simulink model "mup_rmpcblock_demo_model_R2011b"  (Simulink 7.8)
settings: Solver=ode4  StartTime=0.0  StopTime=25  RelTol=1e-3
values from neighbouring files (symbols this model uses):
  A = model.A    [feas_init.m]    (also in mup_expand_rmpc_block_ws.m)
  B = model.B    [feas_init.m]    (also in mup_expand_rmpc_block_ws.m)
  C = model.C    [feas_init.m]    (also in mup_expand_rmpc_block_ws.m)
  nu = size(B{1},2)    [feas_init.m]    (also in mup_expand_rmpc_block_ws.m = problem.nu; mup_rmpcblock_demo.m; mup_sdp.m = problem.nu; rmpc_plot.m = size(data.u{1},1))
  nx = size(A{1},2)    [feas_init.m]    (also in mup_expand_rmpc_block_ws.m = problem.nx; mup_rmpcblock_demo.m; mup_sdp.m = problem.nx; rmpc_plot.m = size(data.x{1},1))
  ts = in(end)    [mup_rmpc_controller.m]    (also in mup_rmpc_counter.m = x(2); mup_rmpcblock_demo.m = 1; rmpc_plot.m = data.ts; rmpc_plot_r13b.m = data.ts)
  u_max = design.u_max    [feas_init.m]    (also in mup_expand_rmpc_block_ws.m; mup_rmpc_demo.m = [10]; mup_rmpcblock_demo.m = [10])
  Wu = design.Wu    [feas_init.m]    (also in mup_expand_rmpc_block_ws.m; mup_rmpc_demo.m = eye(1); mup_rmpcblock_demo.m = eye(1))
  Wx = design.Wx    [feas_init.m]    (also in mup_expand_rmpc_block_ws.m; mup_rmpc_demo.m = eye(2); mup_rmpcblock_demo.m = eye(2))
  x0 = design.x0    [mup_expand_rmpc_block_ws.m]    (also in mup_rmpc_demo.m = [3;0]; mup_rmpcblock_demo.m = [3;0])
  x_max = design.x_max    [feas_init.m]    (also in mup_expand_rmpc_block_ws.m; mup_rmpc_demo.m = [10;10]; mup_rmpcblock_demo.m = [10;10])
settings Model: Creator=oravec  LastModifiedBy=oravec
settings DataIOCC: SignalLoggingSaveFormat=Dataset
settings OptimizationCC: ExpressionDepthLimit=128
settings CodeAppCC: CustomSymbolStrType=$N$R$M_T
settings GRTTargetCC: TargetFunctionLibrary=C89/C90 (ANSI)

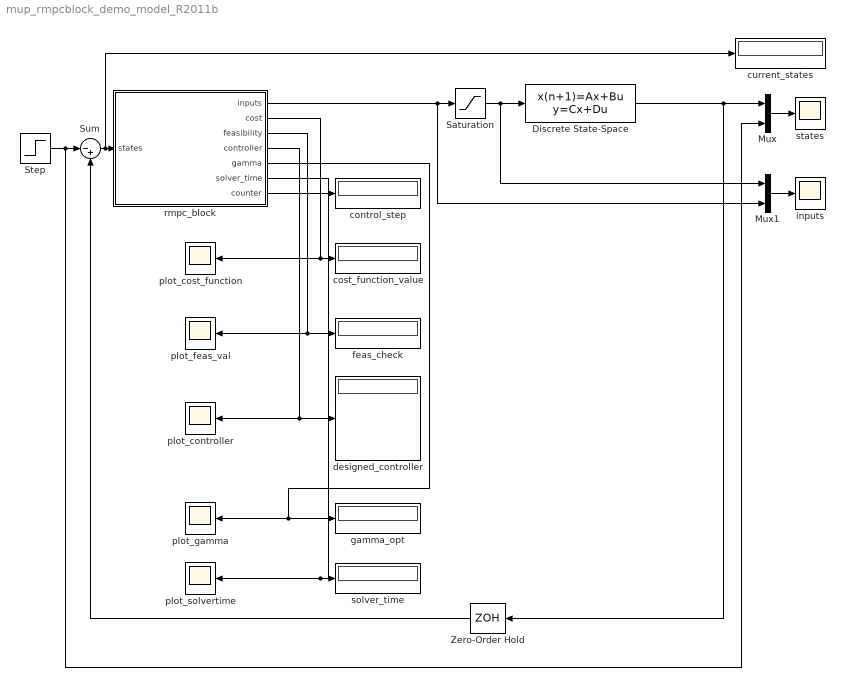
== system mup_rmpcblock_demo_model_R2011b ==
  Discrete State-Space : DiscreteStateSpace  A=A{vtx}  B=B{vtx}  C=C{vtx}  D=zeros(nx,nu)  X0=x0  SampleTime=ts
  Mux : Mux  Inputs=2
  Mux1 : Mux  Inputs=2
  Saturation : Saturate  UpperLimit=u_max  LowerLimit=-u_max
  Step : Step  Time=0  Before=zeros(nx,1)  After=zeros(nx,1)  SampleTime=0
  Sum : Sum  Inputs=|-+
  Zero-Order Hold : ZeroOrderHold  SampleTime=ts
  control_step : Display
  cost_function_value : Display
  current_states : Display
  designed_controller : Display
  feas_check : Display
  gamma_opt : Display
  inputs : Scope
      settings: YMin=-1.1  YMax=0.3  SaveName=data_u
  plot_controller : Scope
      settings: YMin=0  YMax=2  SaveName=f_des
  plot_cost_function : Scope
      settings: YMin=0  YMax=2  SaveName=cost
  plot_feas_val : Scope
      settings: YMin=0  YMax=2  SaveName=feas_val
  plot_gamma : Scope
      settings: YMin=0  YMax=2  SaveName=gamma_val
  plot_solvertime : Scope
      settings: YMin=0  YMax=2  SaveName=solvertime_val
  rmpc_block : Subsystem  Tag=rmpc_tag  mask(RMPC){rmpc_method=Kothare et al. (1996), opt_type=initial, chk_feas=on, feas_toler=-1e-6, x0=x0, A=A, B=B, C=C, Ts=ts, Wu=Wu, Wx=Wx, u_max=u_max, x_max=x_max, param=[], chk_soft_con=off, u_sl=[], y_sl=[], Wsu=[], Wsy=[], solver=MOSEK, vbs=Normal, vbsy=Silent}
      mask prompts: rmpc_method "Robust MPC Approach:"; opt_type "Optimization Problem Design:"; chk_feas "Feasibility Check (Disable to speed up control)"; feas_toler "Feasibility Tolerance: (Relevant, if Feasibility Check is enable)"; x0 "Initial Conditions of System States: x0"; A "System State Matrix: A"; B "System Input Matrix: B"; C "System Output Matrix: C"; Ts "Sampling Time: Ts"; Wu "Cost Function Weight of Inputs: Wu"; Wx "Cost Function Weight of States: Wx"; u_max "Symmetric Constraint on Control Input: u_max"; x_max "Symmetric Constraint on System Outputs: y_max"; param "Parameters:"; chk_soft_con "Consider Soft Constraints: chk_soft_con"; u_sl "Soft-constrained Control Inputs: u_sl"; y_sl "Soft-constrained System Outputs: y_sl"; Wsu "Weight of Soft-constrained Control Inputs: Wsu"; Wsy "Weight of Soft-constrained System Outputs: Wsy"; solver "SDP Solver:"; vbs "Verbose Mode:"; vbsy "YALMIP Verbose Mode:"
      mask help: Computes on-line robust MPC control inputs for a given state.
      mask init:
      | mup_rmpc_data
      | mup_rmpc_init(design,model,setup)
      mask Help: eval('mup_rmpc_help')
      mask StyleString: popup(Kothare et al. (1996)|Cuzzola et al. (2002)|Mao (2003)|Wan et al. (2003)|Cao et al. (2005)|Ding et al. (2007)|Li et al. (2008)|Huang et al. (2011)|Zhang et al. (2013)|NSO and ACIS|NSO and WACIS|NSO and SDLF|PDLF and ACIS|PDLF and WACIS|Kothare et al. (1996) - Soft-Con|Wan et al. (2003) - Soft-Con|Cao et al. (2005) - Soft-Con|NSO and ACIS - Soft-Con),popup(initial|reformulation),checkbox,edit,edit,edit,edit,edit,edit,edit,edit,edit,edit,edit,checkbox,edit,edit,edit,edit,popup(CSDP|DSDP|LMILAB|LOGDETPPA|MOSEK|PENBMI|PENLAB|PENSDP|SDPA|SDPLR|SDPT3|SDPNAL|SEDUMI),popup(Normal|Silent|Loud),popup(Silent|Loud)
      mask TabNameString: Robust MPC Configuration,Robust MPC Configuration,Robust MPC Configuration,Robust MPC Configuration,Robust MPC Configuration,Robust MPC Configuration,Robust MPC Configuration,Robust MPC Configuration,Robust MPC Configuration,Robust MPC Configuration,Robust MPC Configuration,Robust MPC Configuration,Robust MPC Configuration,Robust MPC Configuration,SOFT-CON,SOFT-CON,SOFT-CON,SOFT-CON,SOFT-CON,Setup,Setup,Setup
      mask Display:
      | disp('RMPC')
      | port_label('input',1,'states')
      | port_label('output',1,'inputs')
      | port_label('output',2,'cost')
      | port_label('output',3,'feasibility')
      | port_label('output',4,'controller')
      | port_label('output',5,'gamma')
      | port_label('output',6,'solver_time')
      | port_label('output',7,'counter')
  solver_time : Display
  states : Scope
      settings: YMin=-0.02  YMax=0.1  SaveName=data_x
  wires:
  rmpc_block/2(cost) -> plot_cost_function/1, cost_function_value/1
  Sum/1 -> rmpc_block/1(states), current_states/1
  Step/1 -> Mux/2, Sum/1
  Discrete State-Space/1 -> Mux/1, Zero-Order Hold/1
  Zero-Order Hold/1 -> Sum/2
  Mux/1 -> states/1
  Saturation/1 -> Discrete State-Space/1, Mux1/1
  rmpc_block/1(inputs) -> Saturation/1, Mux1/2
  Mux1/1 -> inputs/1
  rmpc_block/7(counter) -> control_step/1
  rmpc_block/3(feasibility) -> feas_check/1, plot_feas_val/1
  rmpc_block/4(controller) -> designed_controller/1, plot_controller/1
  rmpc_block/5(gamma) -> gamma_opt/1, plot_gamma/1
  rmpc_block/6(solver_time) -> plot_solvertime/1, solver_time/1

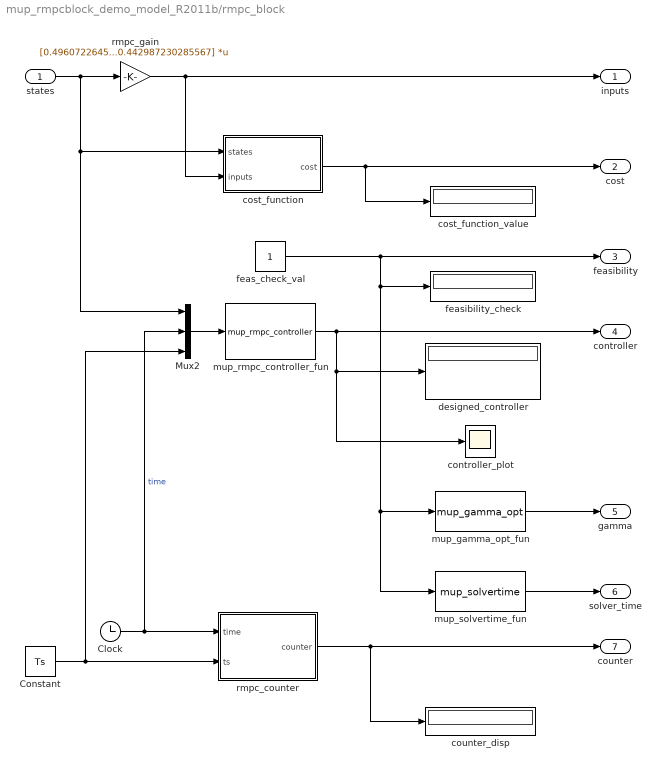
== system mup_rmpcblock_demo_model_R2011b/rmpc_block ==
  states : Inport
  Clock : Clock
  Constant : Constant  Value=Ts
  Mux2 : Mux  Inputs=3
  controller_plot : Scope
      settings: TimeRange=50  SaveName=rmpc_designed_controller  MaxDataPoints=50000
  cost_function : Subsystem
  cost_function_value : Display
  counter_disp : Display
  designed_controller : Display
  feas_check_val : Constant
  feasibility_check : Display
  mup_gamma_opt_fun : MATLABFcn  MATLABFcn=mup_gamma_opt
  mup_rmpc_controller_fun : MATLABFcn  MATLABFcn=mup_rmpc_controller
  mup_solvertime_fun : MATLABFcn  MATLABFcn=mup_solvertime
  rmpc_counter : Subsystem
  rmpc_gain : Gain  Tag=rmpc_gain_2013_3_25_11_17_59.8099  Gain=[0.496072264545493,0.442987230285567]  Multiplication=Matrix(K*u)
  inputs : Outport
  cost : Outport  Port=2
  feasibility : Outport  Port=3
  controller : Outport  Port=4
  gamma : Outport  Port=5
  solver_time : Outport  Port=6
  counter : Outport  Port=7
  wires:
  rmpc_gain/1 -> inputs/1, cost_function/2(inputs)
  states/1 -> rmpc_gain/1, Mux2/1, cost_function/1(states)
  cost_function/1(cost) -> cost_function_value/1, cost/1
  rmpc_counter/1(counter) -> counter_disp/1, counter/1
  Clock/1 -> rmpc_counter/1(time), Mux2/2  "time"
  Constant/1 -> rmpc_counter/2(ts), Mux2/3
  feas_check_val/1 -> feasibility/1, mup_solvertime_fun/1, mup_gamma_opt_fun/1, feasibility_check/1
  mup_rmpc_controller_fun/1 -> controller/1, designed_controller/1, controller_plot/1
  Mux2/1 -> mup_rmpc_controller_fun/1
  mup_gamma_opt_fun/1 -> gamma/1
  mup_solvertime_fun/1 -> solver_time/1

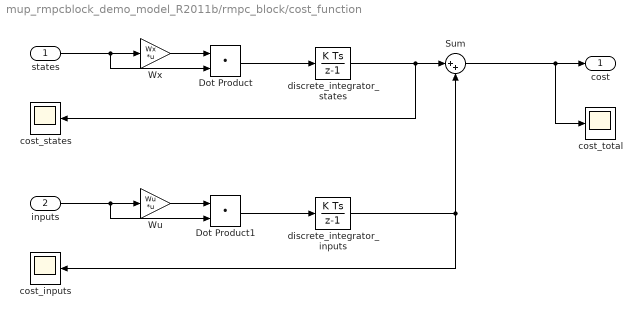
== system mup_rmpcblock_demo_model_R2011b/rmpc_block/cost_function ==
  states : Inport
  inputs : Inport  Port=2
  Dot Product : DotProduct  InputSameDT=on  OutDataTypeStr=Inherit: Inherit via internal rule
  Dot Product1 : DotProduct  InputSameDT=on  OutDataTypeStr=Inherit: Inherit via internal rule
  Sum : Sum  Inputs=|++
  Wu : Gain  Gain=Wu  Multiplication=Matrix(K*u)
  Wx : Gain  Gain=Wx  Multiplication=Matrix(K*u)
  cost_inputs : Scope
  cost_states : Scope
      settings: SaveName=ScopeData2
  cost_total : Scope
      settings: SaveName=ScopeData3
  discrete_integrator_inputs : DiscreteIntegrator  SampleTime=Ts
  discrete_integrator_states : DiscreteIntegrator  SampleTime=Ts
  cost : Outport
  wires:
  Dot Product1/1 -> discrete_integrator_inputs/1
  Wu/1 -> Dot Product1/1
  Dot Product/1 -> discrete_integrator_states/1
  Wx/1 -> Dot Product/1
  states/1 -> Dot Product/2, Wx/1
  inputs/1 -> Dot Product1/2, Wu/1
  Sum/1 -> cost/1, cost_total/1
  discrete_integrator_states/1 -> Sum/1, cost_states/1
  discrete_integrator_inputs/1 -> Sum/2, cost_inputs/1

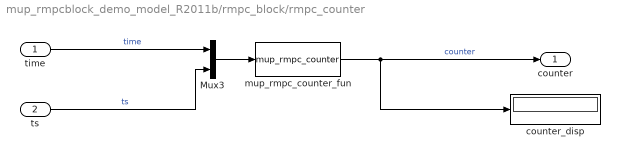
== system mup_rmpcblock_demo_model_R2011b/rmpc_block/rmpc_counter ==
  time : Inport
  ts : Inport  Port=2
  Mux3 : Mux  Inputs=2
  counter_disp : Display
  mup_rmpc_counter_fun : MATLABFcn  MATLABFcn=mup_rmpc_counter
  counter : Outport
  wires:
  mup_rmpc_counter_fun/1 -> counter/1, counter_disp/1  "counter"
  ts/1 -> Mux3/2  "ts"
  time/1 -> Mux3/1  "time"
  Mux3/1 -> mup_rmpc_counter_fun/1
